simulink model "Neurofeedback_PID_WithoutFNIRS_v1"  (R2021b)
settings: Solver=VariableStepAuto  StartTime=0.0  StopTime=60  FixedStep=0.09  RelTol=1e-10
libraries: slpidlib x1
settings Model: NumberOfSteps=10  SnapshotInterval=100  Creator=mdls3  LastModifiedBy=mdls3
settings SolverCC: ZeroCrossControl=EnableAll
settings DebuggingCC: UnderSpecifiedDimensionMsg=warning

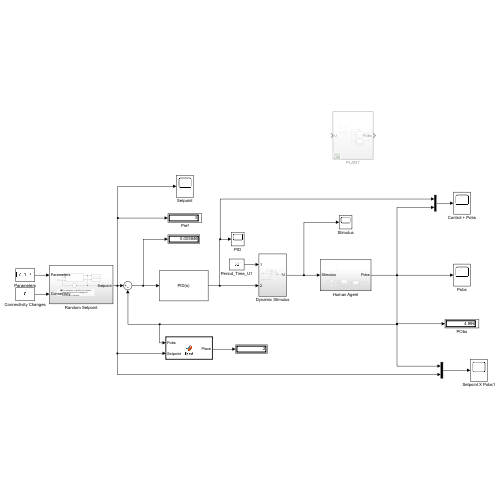
[thumbnail: Simulink's stored preview of the top-level diagram]
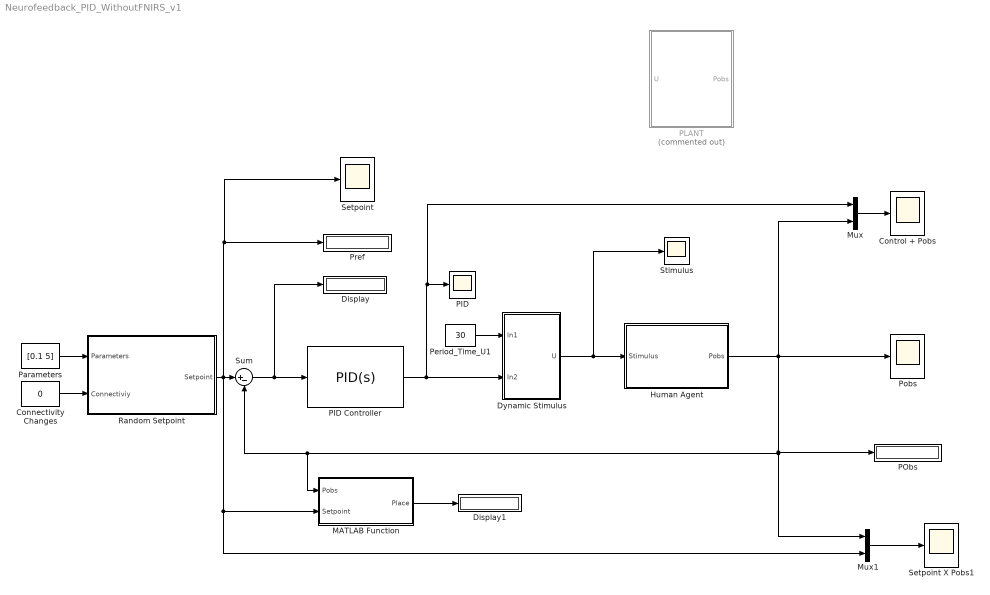
== system Neurofeedback_PID_WithoutFNIRS_v1 ==
  Connectivity Changes : Constant  Value=0
  Control + Pobs : Scope
  Display : Display
  Display1 : Display
  Dynamic Stimulus : Subsystem
  Human Agent : Subsystem
  MATLAB Function : MATLAB Function  TreatAsAtomicUnit=on
  Mux : Mux  Inputs=2
  Mux1 : Mux  Inputs=2
  PID : Scope
  PID Controller : slpidlib/PID Controller  Controller=PID  Form=Ideal  TimeDomain=Continuous-time  UseExternalTs=off  SampleTime=-1  IntegratorMethod=Forward Euler  FilterMethod=Forward Euler  ControllerParametersSource=internal  P=0.6  I=0.075  D=0.015  UseFilter=on  N=100  TunerSelectOption=Transfer Function Based (PID Tuner App)  InitialConditionSource=internal  InitialConditionForIntegrator=1  InitialConditionForFilter=0  DifferentiatorICPrevScaledInput=0  ExternalReset=none  TrackingMode=off  Kt=1  LimitOutput=off  SatLimitsSource=internal  UpperSaturationLimit=inf  LowerSaturationLimit=-inf  LinearizeAsGain=on  AntiWindupMode=none  Kb=1  POutMin=[]  POutMax=[]  IOutMin=[]  IOutMax=[]  DOutMin=[]  DOutMax=[]  NOutMin=[]  NOutMax=[]  SumOutMin=[]  SumOutMax=[]  SaturationOutMin=[]  SaturationOutMax=[]  PParamMin=[]  PParamMax=[]  IParamMin=[]  IParamMax=[]  DParamMin=[]  DParamMax=[]  NParamMin=[]  NParamMax=[]  KbParamMin=[]  KbParamMax=[]  KtParamMin=[]  KtParamMax=[]  KbOutMin=[]  KbOutMax=[]  KtOutMin=[]  KtOutMax=[]  IntegratorOutMin=[]  IntegratorOutMax=[]  FilterOutMin=[]  FilterOutMax=[]  SumI1OutMin=[]  SumI1OutMax=[]  SumI2OutMin=[]  SumI2OutMax=[]  SumI3OutMin=[]  SumI3OutMax=[]  SumI4OutMin=[]  SumI4OutMax=[]  SumDOutMin=[]  SumDOutMax=[]  DifferentiatorOutMin=[]  DifferentiatorOutMax=[]  FilterDiffOutCoefMin=[]  FilterDiffOutCoefMax=[]  ReciprocalOutMin=[]  ReciprocalOutMax=[]  SumDenOutMin=[]  SumDenOutMax=[]  SumNumOutMin=[]  SumNumOutMax=[]  DivideOutMin=[]  DivideOutMax=[]  UdiffTsProdOutMin=[]  UdiffTsProdOutMax=[]  NTsProdOutMin=[]  NTsProdOutMax=[]  UintegralTsProdOutMin=[]  UintegralTsProdOutMax=[]  UngainTsProdOutMin=[]  UngainTsProdOutMax=[]  IntegratorContinuousStateAttributes=''  IntegratorStateMustResolveToSignalObject=off  IntegratorRTWStateStorageClass=Auto  FilterContinuousStateAttributes=''  FilterStateMustResolveToSignalObject=off  FilterRTWStateStorageClass=Auto  ParallelPVariant=Passthrough  IdealPVariant=InternalParameters  IVariant=InternalParameters  DVariant=InternalParameters  IntegratorVariant=Continuous  SatVariant=Disabled  AWVariant=Passthrough  PCopyVariant=Disabled  TRVariant=Disabled  FdbkBlocksVariant=Forward  IdealPFdbkVariant=Disabled  SatFdbkVariant=Disabled  DerivativeFilterVariant=ContFilter  NVariant=InternalParameters  NCopyVariant=Disabled  FilterICVariant=InternalICsFilter  IntegratorICVariant=InternalICs  ExternalResetVariant=Disabled  TRSumVariant=Passthrough  SumFdbkVariant=Disabled  SumVariant=Sum_PID  TsampFilterVariant=InternalTs  TsampNgainVariant=Passthrough  TsampIntegralVariant=Passthrough  ExternalSaturationOutDataTypeStr=Inherit: Same as second input
  PLANT : Subsystem  Commented=on
  PObs : Display
  Parameters : Constant  Value=[0.1 5]
  Period_Time_U1 : Constant  Value=30
  Pobs : Scope
  Pref : Display
  Random Setpoint : Subsystem
  Setpoint : Scope
  Setpoint X Pobs1 : Scope
  Stimulus : Scope
  Sum : Sum  Inputs=|+-
  wires:
  Period_Time_U1/1 -> Dynamic Stimulus/1(In1)
  Dynamic Stimulus/1(U) -> Stimulus/1, Human Agent/1(Stimulus)
  PID Controller/1 -> Dynamic Stimulus/2(In2), Mux/1, PID/1
  Sum/1 -> PID Controller/1, Display/1
  Human Agent/1(Pobs) -> Mux1/1, MATLAB Function/1(Pobs), Sum/2, PObs/1, Pobs/1, Mux/2
  Parameters/1 -> Random Setpoint/1(Parameters)
  Random Setpoint/1(Setpoint) -> MATLAB Function/2(Setpoint), Mux1/2, Setpoint/1, Pref/1, Sum/1
  Connectivity Changes/1 -> Random Setpoint/2(Connectiviy)
  Mux/1 -> Control + Pobs/1
  Mux1/1 -> Setpoint X Pobs1/1
  MATLAB Function/1(Place) -> Display1/1

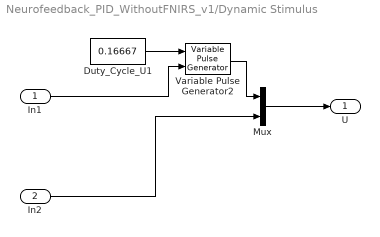
== system Neurofeedback_PID_WithoutFNIRS_v1/Dynamic Stimulus ==
  In1 : Inport
  In2 : Inport  Port=2
  Duty_Cycle_U1 : Constant  Value=0.16667  OutMin=[0]  OutMax=[0.8]
  Mux : Mux  Inputs=2
  Variable Pulse Generator2 : VariablePulseGenerator  RunAtFixedTimeIntervals=on  SampleTime=1/10.4
  U : Outport
  wires:
  In1/1 -> Variable Pulse Generator2/2
  Mux/1 -> U/1
  Variable Pulse Generator2/1 -> Mux/1
  Duty_Cycle_U1/1 -> Variable Pulse Generator2/1
  In2/1 -> Mux/2

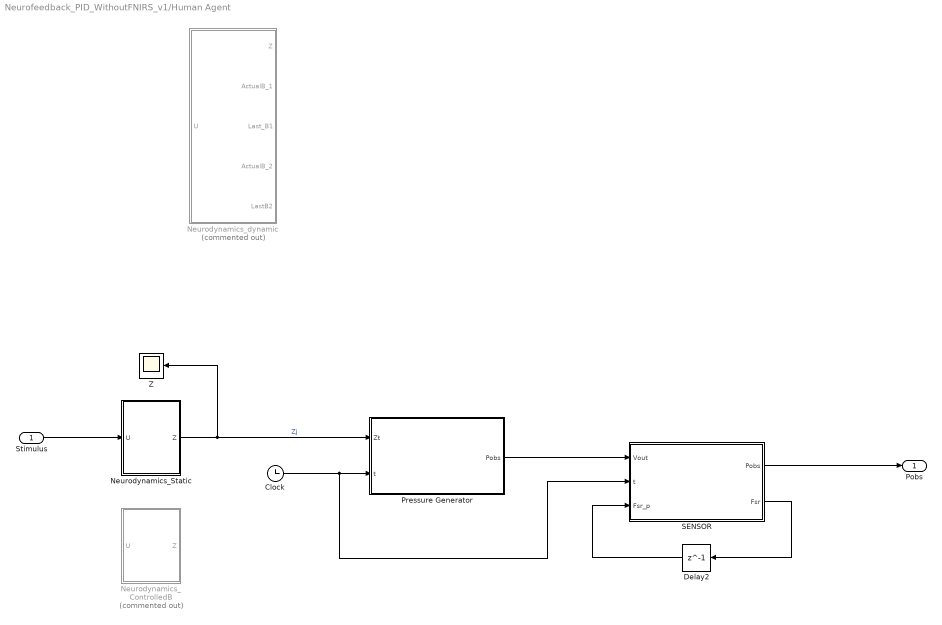
== system Neurofeedback_PID_WithoutFNIRS_v1/Human Agent ==
  Stimulus : Inport
  Clock : Clock
  Delay2 : Delay  DelayLength=1  InitialCondition=0.0001
  Neurodynamics_ControlledB : Subsystem  Commented=on
  "Neurodynamics_Static " : Subsystem
  Neurodynamics_dynamic : Subsystem  Commented=on
  Pressure Generator : MATLAB Function  TreatAsAtomicUnit=on
  SENSOR : MATLAB Function  TreatAsAtomicUnit=on
  Z : Scope
  Pobs : Outport
  wires:
  Pressure Generator/1(Pobs) -> SENSOR/1(Vout)
  Delay2/1 -> SENSOR/3(Fsr_p)
  SENSOR/2(Fsr) -> Delay2/1
  SENSOR/1(Pobs) -> Pobs/1
  Clock/1 -> Pressure Generator/2(t), SENSOR/2(t)
  "Neurodynamics_Static "/1(Z) -> Pressure Generator/1(Zt), Z/1  "Zj"
  Stimulus/1 -> "Neurodynamics_Static "/1(U)

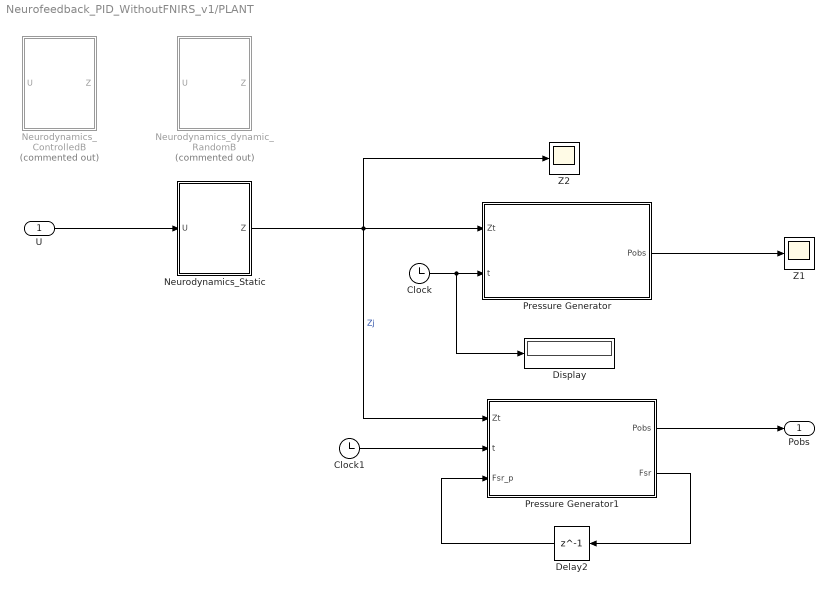
== system Neurofeedback_PID_WithoutFNIRS_v1/PLANT ==
  U : Inport
  Clock : Clock
  Clock1 : Clock
  Delay2 : Delay  DelayLength=1  InitialCondition=0.0001
  Display : Display
  Neurodynamics_ControlledB : Subsystem  Commented=on
  "Neurodynamics_Static " : Subsystem
  Neurodynamics_dynamic_RandomB : Subsystem  Commented=on
  Pressure Generator : MATLAB Function  TreatAsAtomicUnit=on
  Pressure Generator1 : MATLAB Function  TreatAsAtomicUnit=on
  Z1 : Scope
  Z2 : Scope
  Pobs : Outport
  wires:
  Clock/1 -> Display/1, Pressure Generator/2(t)
  Clock1/1 -> Pressure Generator1/2(t)
  Pressure Generator1/2(Fsr) -> Delay2/1
  Pressure Generator1/1(Pobs) -> Pobs/1
  Delay2/1 -> Pressure Generator1/3(Fsr_p)
  Pressure Generator/1(Pobs) -> Z1/1
  "Neurodynamics_Static "/1(Z) -> Pressure Generator1/1(Zt), Z2/1, Pressure Generator/1(Zt)  "Zj"
  U/1 -> "Neurodynamics_Static "/1(U)

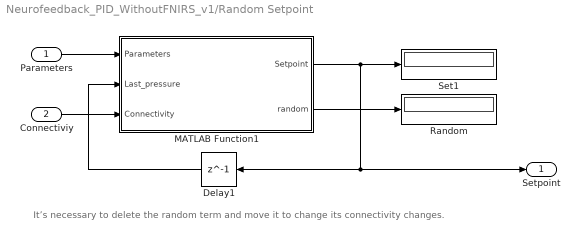
== system Neurofeedback_PID_WithoutFNIRS_v1/Random Setpoint ==
  note: It’s necessary to delete the random term and move it to change its connectivity changes.
  Parameters : Inport
  Connectiviy : Inport  Port=2
  Delay1 : Delay  DelayLength=1  InitialCondition=0
  MATLAB Function1 : MATLAB Function  TreatAsAtomicUnit=on
  Random : Display
  Set1 : Display
  Setpoint : Outport
  wires:
  Parameters/1 -> MATLAB Function1/1(Parameters)
  MATLAB Function1/2(random) -> Random/1
  MATLAB Function1/1(Setpoint) -> Set1/1, Setpoint/1, Delay1/1
  Delay1/1 -> MATLAB Function1/2(Last_pressure)
  Connectiviy/1 -> MATLAB Function1/3(Connectivity)

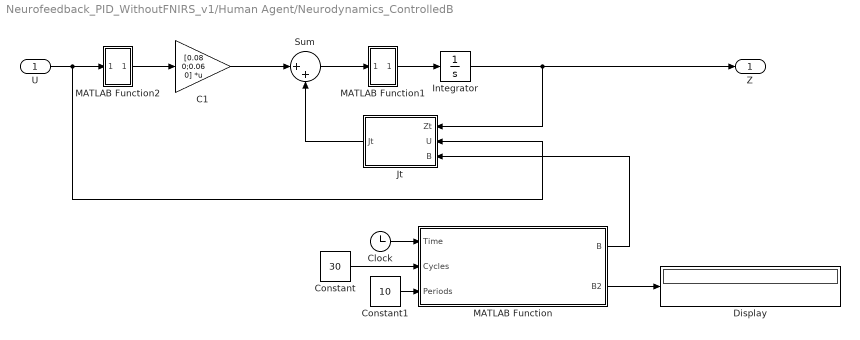
== system Neurofeedback_PID_WithoutFNIRS_v1/Human Agent/Neurodynamics_ControlledB ==
  U : Inport
  C1 : Gain  Gain=[0.08 0;0.06 0]  Multiplication=Matrix(K*u) (u vector)
  Clock : Clock
  Constant : Constant  Value=30
  Constant1 : Constant  Value=10
  Display : Display
  Integrator : Integrator
  Jt : MATLAB Function  TreatAsAtomicUnit=on
  MATLAB Function : MATLAB Function  TreatAsAtomicUnit=on
  MATLAB Function1 : MATLAB Function  TreatAsAtomicUnit=on
  MATLAB Function2 : MATLAB Function  TreatAsAtomicUnit=on
  Sum : Sum  Inputs=|++
  Z : Outport
  wires:
  Jt/1(Jt) -> Sum/2
  U/1 -> MATLAB Function2/1(Z), Jt/2(U)
  Constant1/1 -> MATLAB Function/3(Periods)
  Clock/1 -> MATLAB Function/1(Time)
  Constant/1 -> MATLAB Function/2(Cycles)
  MATLAB Function/2(B2) -> Display/1
  MATLAB Function/1(B) -> Jt/3(B)
  Integrator/1 -> Z/1, Jt/1(Zt)
  MATLAB Function1/1(Zn) -> Integrator/1
  Sum/1 -> MATLAB Function1/1(Z)
  MATLAB Function2/1(Zn) -> C1/1
  C1/1 -> Sum/1

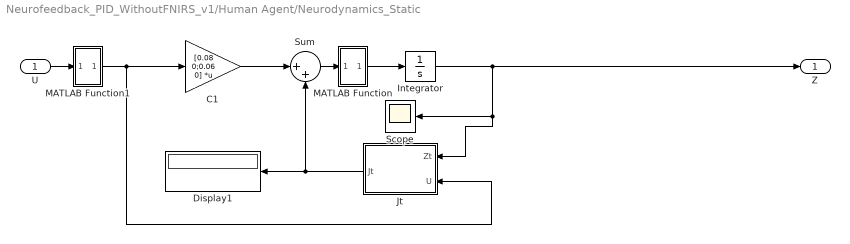
== system Neurofeedback_PID_WithoutFNIRS_v1/Human Agent/Neurodynamics_Static  ==
  U : Inport
  C1 : Gain  Gain=[0.08 0;0.06 0]  Multiplication=Matrix(K*u) (u vector)
  Display1 : Display
  Integrator : Integrator
  Jt : MATLAB Function  TreatAsAtomicUnit=on
  MATLAB Function : MATLAB Function  TreatAsAtomicUnit=on
  MATLAB Function1 : MATLAB Function  TreatAsAtomicUnit=on
  Scope : Scope
  Sum : Sum  Inputs=|++
  Z : Outport
  wires:
  Integrator/1 -> Z/1, Scope/1, Jt/1(Zt)
  C1/1 -> Sum/1
  Jt/1(Jt) -> Sum/2, Display1/1
  U/1 -> MATLAB Function1/1(Z)
  Sum/1 -> MATLAB Function/1(Z)
  MATLAB Function1/1(Zn) -> C1/1, Jt/2(U)
  MATLAB Function/1(Zn) -> Integrator/1

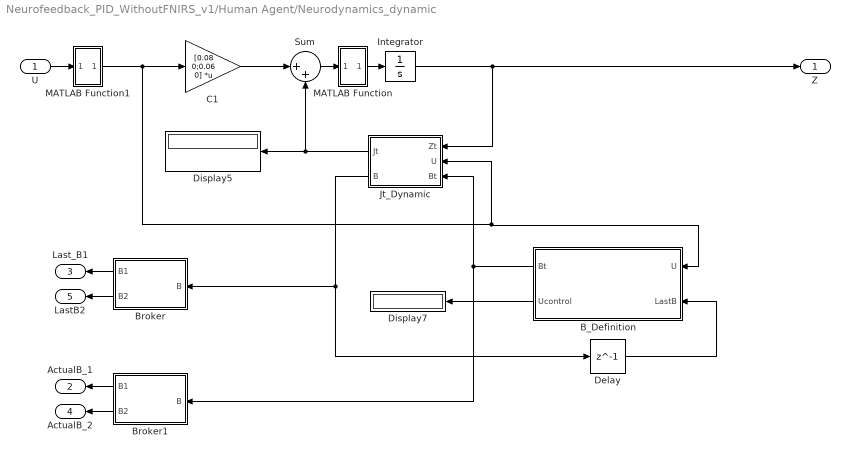
== system Neurofeedback_PID_WithoutFNIRS_v1/Human Agent/Neurodynamics_dynamic ==
  U : Inport
  B_Definition : MATLAB Function  TreatAsAtomicUnit=on
  Broker : MATLAB Function  TreatAsAtomicUnit=on
  Broker1 : MATLAB Function  TreatAsAtomicUnit=on
  C1 : Gain  Gain=[0.08 0;0.06 0]  Multiplication=Matrix(K*u) (u vector)
  Delay : Delay  DelayLength=1  InitialCondition=0
  Display5 : Display
  Display7 : Display
  Integrator : Integrator
  Jt_Dynamic : MATLAB Function  TreatAsAtomicUnit=on
  MATLAB Function : MATLAB Function  TreatAsAtomicUnit=on
  MATLAB Function1 : MATLAB Function  TreatAsAtomicUnit=on
  Sum : Sum  Inputs=|++
  Z : Outport
  ActualB_1 : Outport  Port=2
  Last_B1 : Outport  Port=3
  ActualB_2 : Outport  Port=4
  LastB2 : Outport  Port=5
  wires:
  Integrator/1 -> Z/1, Jt_Dynamic/1(Zt)
  C1/1 -> Sum/1
  U/1 -> MATLAB Function1/1(Z)
  Sum/1 -> MATLAB Function/1(Z)
  MATLAB Function1/1(Zn) -> C1/1, B_Definition/1(U), Jt_Dynamic/2(U)
  MATLAB Function/1(Zn) -> Integrator/1
  Jt_Dynamic/1(Jt) -> Display5/1, Sum/2
  Delay/1 -> B_Definition/2(LastB)
  Jt_Dynamic/2(B) -> Broker/1(B), Delay/1
  B_Definition/1(Bt) -> Jt_Dynamic/3(Bt), Broker1/1(B)
  B_Definition/2(Ucontrol) -> Display7/1
  Broker1/1(B1) -> ActualB_1/1
  Broker1/2(B2) -> ActualB_2/1
  Broker/2(B2) -> LastB2/1
  Broker/1(B1) -> Last_B1/1

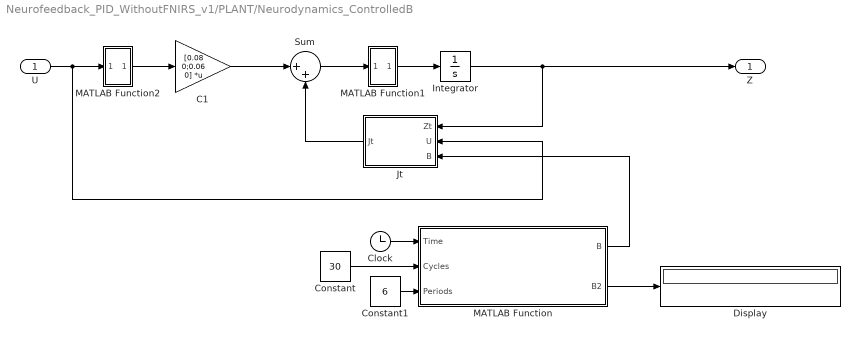
== system Neurofeedback_PID_WithoutFNIRS_v1/PLANT/Neurodynamics_ControlledB ==
  U : Inport
  C1 : Gain  Gain=[0.08 0;0.06 0]  Multiplication=Matrix(K*u) (u vector)
  Clock : Clock
  Constant : Constant  Value=30
  Constant1 : Constant  Value=6
  Display : Display
  Integrator : Integrator
  Jt : MATLAB Function  TreatAsAtomicUnit=on
  MATLAB Function : MATLAB Function  TreatAsAtomicUnit=on
  MATLAB Function1 : MATLAB Function  TreatAsAtomicUnit=on
  MATLAB Function2 : MATLAB Function  TreatAsAtomicUnit=on
  Sum : Sum  Inputs=|++
  Z : Outport
  wires:
  Jt/1(Jt) -> Sum/2
  U/1 -> MATLAB Function2/1(Z), Jt/2(U)
  Constant1/1 -> MATLAB Function/3(Periods)
  Clock/1 -> MATLAB Function/1(Time)
  Constant/1 -> MATLAB Function/2(Cycles)
  MATLAB Function/2(B2) -> Display/1
  MATLAB Function/1(B) -> Jt/3(B)
  Integrator/1 -> Z/1, Jt/1(Zt)
  MATLAB Function1/1(Zn) -> Integrator/1
  Sum/1 -> MATLAB Function1/1(Z)
  MATLAB Function2/1(Zn) -> C1/1
  C1/1 -> Sum/1

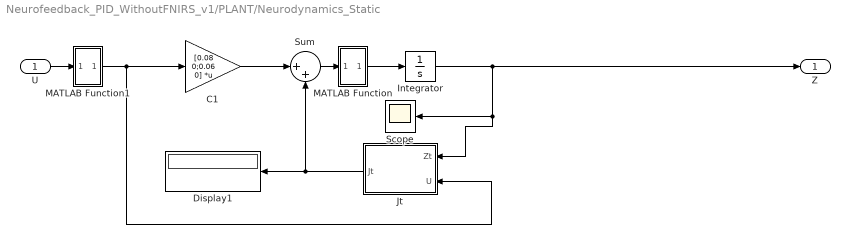
== system Neurofeedback_PID_WithoutFNIRS_v1/PLANT/Neurodynamics_Static  ==
  U : Inport
  C1 : Gain  Gain=[0.08 0;0.06 0]  Multiplication=Matrix(K*u) (u vector)
  Display1 : Display
  Integrator : Integrator
  Jt : MATLAB Function  TreatAsAtomicUnit=on
  MATLAB Function : MATLAB Function  TreatAsAtomicUnit=on
  MATLAB Function1 : MATLAB Function  TreatAsAtomicUnit=on
  Scope : Scope
  Sum : Sum  Inputs=|++
  Z : Outport
  wires:
  Integrator/1 -> Z/1, Scope/1, Jt/1(Zt)
  C1/1 -> Sum/1
  Jt/1(Jt) -> Sum/2, Display1/1
  U/1 -> MATLAB Function1/1(Z)
  Sum/1 -> MATLAB Function/1(Z)
  MATLAB Function1/1(Zn) -> C1/1, Jt/2(U)
  MATLAB Function/1(Zn) -> Integrator/1

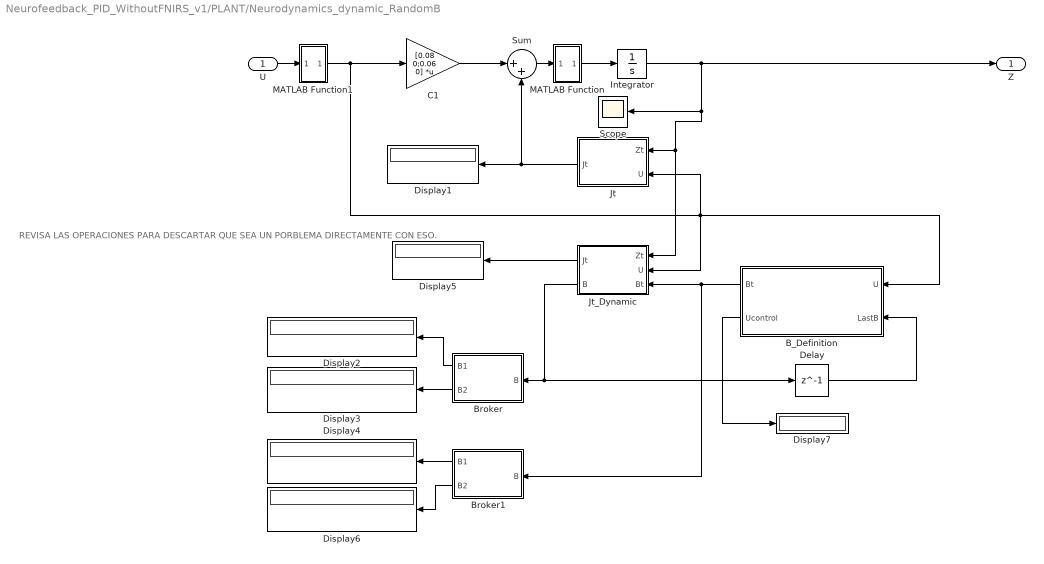
== system Neurofeedback_PID_WithoutFNIRS_v1/PLANT/Neurodynamics_dynamic_RandomB ==
  note: REVISA LAS OPERACIONES PARA DESCARTAR QUE SEA UN PORBLEMA DIRECTAMENTE CON ESO.
  U : Inport
  B_Definition : MATLAB Function  TreatAsAtomicUnit=on
  Broker : MATLAB Function  TreatAsAtomicUnit=on
  Broker1 : MATLAB Function  TreatAsAtomicUnit=on
  C1 : Gain  Gain=[0.08 0;0.06 0]  Multiplication=Matrix(K*u) (u vector)
  Delay : Delay  DelayLength=1  InitialCondition=0
  Display{1..7} (7 alike) : Display
  Integrator : Integrator
  Jt : MATLAB Function  TreatAsAtomicUnit=on
  Jt_Dynamic : MATLAB Function  TreatAsAtomicUnit=on
  MATLAB Function : MATLAB Function  TreatAsAtomicUnit=on
  MATLAB Function1 : MATLAB Function  TreatAsAtomicUnit=on
  Scope : Scope
  Sum : Sum  Inputs=|++
  Z : Outport
  wires:
  Integrator/1 -> Z/1, Scope/1, Jt/1(Zt), Jt_Dynamic/1(Zt)
  C1/1 -> Sum/1
  Jt/1(Jt) -> Sum/2, Display1/1
  U/1 -> MATLAB Function1/1(Z)
  Sum/1 -> MATLAB Function/1(Z)
  MATLAB Function1/1(Zn) -> C1/1, Jt/2(U), B_Definition/1(U), Jt_Dynamic/2(U)
  MATLAB Function/1(Zn) -> Integrator/1
  Jt_Dynamic/1(Jt) -> Display5/1
  Delay/1 -> B_Definition/2(LastB)
  Jt_Dynamic/2(B) -> Broker/1(B), Delay/1
  Broker/1(B1) -> Display2/1
  Broker/2(B2) -> Display3/1
  B_Definition/1(Bt) -> Broker1/1(B), Jt_Dynamic/3(Bt)
  Broker1/2(B2) -> Display6/1
  Broker1/1(B1) -> Display4/1
  B_Definition/2(Ucontrol) -> Display7/1

== matlab function Neurofeedback_PID_WithoutFNIRS_v1/PLANT/Neurodynamics_dynamic_RandomB/Jt ==
  data: Zt input; U input; Jt output
function Jt = fcn(Zt, U)
   A = [-0.16 -0.49;-0.02 -0.33];
   nRegions  = size(A,1);
   M = size(U,1); %nStimuli
   simulationLength = size(U,2);
   B = zeros(2,2,2);
   B1 = [0 0; 0 0]; %There must be a B per stimulus
   B2 = [-0.02 -0.77; 0.33 -1.31];
   B(:,:,1) = B1;
   B(:,:,2) = B2;
      assert(M == size(B,3),...
       'Unexpected number of induced connectivity parameters B.');
   T = zeros(nRegions); %nRegions x nRegions
    for t = 1:simulationLength
           for uu = 1:M % Sum (Uj * Bj)
               tmp = U(uu,t)*B(:,:,uu);
               T = -0.5*exp(T + tmp);  
           end
    end
    SI = diag(A);
    A =  A - diag(exp(SI) + (SI));
Jt = (A*Zt) + (T*Zt);

== matlab function Neurofeedback_PID_WithoutFNIRS_v1/PLANT/Neurodynamics_ControlledB/Jt ==
  data: Zt input; U input; Jt output; B input
function Jt = fcn(Zt, U,B)
   A = [-0.16 -0.49;-0.02 -0.33];
   nRegions  = size(A,1);
   M = size(U,1); %nStimuli
   simulationLength = size(U,2);
%    B = zeros(2,2,2);
%    B1 = [0 0; 0 0]; %There must be a B per stimulus
%    %B2_3
%    B2 = [-0.67 -0.91 ;-0.3 -1.21];
%    %B2_2
%    %B2 = [-0.08 -1.08; 1.2054 -0.0076];
%    %B2_1
%    %B2 = [-0.02 -0.07; 0.33 -1.31];
%    B(:,:,1) = B1;
%    B(:,:,2) = B2;
      assert(M == size(B,3),...
       'Unexpected number of induced connectivity parameters B.');
   T = zeros(nRegions); %nRegions x nRegions
    for t = 1:simulationLength
           for uu = 1:M % Sum (Uj * Bj)
               tmp = U(uu,t)*B(:,:,uu);
               T = -0.5*exp(T + tmp);  
           end
    end
    SI = diag(A);
    A =  A - diag(exp(SI) + (SI));
Jt = (A*Zt) + (T*Zt);

== matlab function Neurofeedback_PID_WithoutFNIRS_v1/PLANT/Neurodynamics_dynamic_RandomB/MATLAB Function ==
  data: Z input; Zn output
function Zn = fcn(Z)

Zn = Z(:,1);

== matlab function Neurofeedback_PID_WithoutFNIRS_v1/PLANT/Neurodynamics_dynamic_RandomB/MATLAB Function1 ==
  data: Z input; Zn output
function Zn = fcn(Z)

Zn = Z(:,1);

== matlab function Neurofeedback_PID_WithoutFNIRS_v1/Human Agent/Neurodynamics_Static /Jt ==
  data: Zt input; U input; Jt output
function Jt = fcn(Zt, U)
   A = [-0.16 -0.49;-0.02 -0.33];
   nRegions  = size(A,1);
   M = size(U,1); %nStimuli
   simulationLength = size(U,2);
   B = zeros(2,2,2);
   B1 = [0 0; 0 0]; %There must be a B per stimulus
   B2 = [-0.02 -0.77; 0.33 -1.31];
   B(:,:,1) = B1;
   B(:,:,2) = B2;
      assert(M == size(B,3),...
       'Unexpected number of induced connectivity parameters B.');
   T = zeros(nRegions); %nRegions x nRegions
    for t = 1:simulationLength
           for uu = 1:M % Sum (Uj * Bj)
               tmp = U(uu,t)*B(:,:,uu);
               T = -0.5*exp(T + tmp);  
           end
    end
    SI = diag(A);
    A =  A - diag(exp(SI) + (SI));
Jt = (A*Zt) + (T*Zt);

== matlab function Neurofeedback_PID_WithoutFNIRS_v1/PLANT/Pressure Generator ==
  data: Zt input; Pobs output; t input
function Pobs = fcn(Zt, t)
    R=10000; %Resistor [Ohms];
    C=0.1; %Capacitor [Faradays];
    V= Zt(1,:); %Voltage or system reference;
    Vc = V * (1 - exp(-t/(R*C))); % Voltage at the capacitor  
    
Pobs = Vc;

== matlab function Neurofeedback_PID_WithoutFNIRS_v1/Human Agent/Neurodynamics_Static /MATLAB Function ==
  data: Z input; Zn output
function Zn = fcn(Z)

Zn = Z(:,1);

== matlab function Neurofeedback_PID_WithoutFNIRS_v1/Human Agent/Neurodynamics_Static /MATLAB Function1 ==
  data: Z input; Zn output
function Zn = fcn(Z)

Zn = Z(:,1);

== matlab function Neurofeedback_PID_WithoutFNIRS_v1/PLANT/Neurodynamics_Static /Jt ==
  data: Zt input; U input; Jt output
function Jt = fcn(Zt, U)
   A = [-0.16 -0.49;-0.02 -0.33];
   nRegions  = size(A,1);
   M = size(U,1); %nStimuli
   simulationLength = size(U,2);
   B = zeros(2,2,2);
   B1 = [0 0; 0 0]; %There must be a B per stimulus
   B2 = [-0.02 -0.77; 0.33 -1.31];
   B(:,:,1) = B1;
   B(:,:,2) = B2;
      assert(M == size(B,3),...
       'Unexpected number of induced connectivity parameters B.');
   T = zeros(nRegions); %nRegions x nRegions
    for t = 1:simulationLength
           for uu = 1:M % Sum (Uj * Bj)
               tmp = U(uu,t)*B(:,:,uu);
               T = -0.5*exp(T + tmp);  
           end
    end
    SI = diag(A);
    A =  A - diag(exp(SI) + (SI));
Jt = (A*Zt) + (T*Zt);

== matlab function Neurofeedback_PID_WithoutFNIRS_v1/Human Agent/Neurodynamics_ControlledB/MATLAB Function ==
  settings: updateMethod=DISCRETE
  data: Time input; B output; Cycles input; Periods input; B2 output
function [B, B2] = ControlledDynamic_B(Time, Cycles, Periods)

   B = zeros(2,2,2);
   %B1 = [0 0; 0 0]; %There must be a B per stimulus
   %B2_3
   %B2 = [-0.67 -0.91 ;-0.3 -1.21];
   %B2_2
   %B2 = [-0.08 -1.08; 1.2054 -0.0076];
   %B2_1
   %B2 = [-0.02 -0.07; 0.33 -1.31];
   PCycles = zeros(10,1);
   for i = 1:Periods
       PCycles(i) = i * Cycles;   
   end
   %random_selector = randi([1,3]);

   if(Time >= 0 && Time <= PCycles(2))
%       random_selector = randi([1,3]);
%       if(random_selector == 1)
          B1 = [0 0; 0 0];
          B2 = [-0.02 -0.07; 0.33 -1.31]; 
%       elseif(random_selector == 2)
%           B1 = [0 0; 0 0];
%           B2 = [-0.08 -1.08; 1.2054 -0.0076];
%       else
%           B1 = [0 0; 0 0];
%           B2 = [-0.67 -0.91; 0.3 -1.21];
      B(:,:,1) = B1;
      B(:,:,2) = B2;
   elseif(Time >= PCycles(2)+1 && Time <= PCycles(4))
       B1 = [0 0;0 0];
       B2 = [-0.08 -1.08; 1.2054 -0.0076];
       B(:,:,1) = B1;
       B(:,:,2) = B2;
   else
       B1 = [0 0; 0 0];
       B2 = [-0.67 -0.91; -0.3 -1.21];
       B(:,:,1) = B1;
       B(:,:,2) = B2;
   end

== matlab function Neurofeedback_PID_WithoutFNIRS_v1/PLANT/Neurodynamics_Static /MATLAB Function ==
  data: Z input; Zn output
function Zn = fcn(Z)

Zn = Z(:,1);

== matlab function Neurofeedback_PID_WithoutFNIRS_v1/PLANT/Neurodynamics_Static /MATLAB Function1 ==
  data: Z input; Zn output
function Zn = fcn(Z)

Zn = Z(:,1);

== matlab function Neurofeedback_PID_WithoutFNIRS_v1/MATLAB Function ==
  data: Pobs input; Place output; Setpoint input
function Place = feed(Pobs, Setpoint)
    
    %Sensor maximum limit 
    Range = 10;
    Limit =  (Range - Setpoint)/2;
    temp = 0;
    Nm = (Setpoint - Limit);
    Nl = (Setpoint - Limit)*2;
    
    Pl = (Setpoint + Limit);
    Pm = (Setpoint + Limit)*2;
    
    if ((Pobs > Pl) && (Pobs < Pm))
        temp = 4;
    elseif((Pobs > Setpoint) && (Pobs < Pl))
        temp = 3;
    elseif((Pobs > Nm) && (Pobs < Setpoint))
        temp = 2;
    else
        temp = 1;

    end
    
    Place = temp;

== matlab function Neurofeedback_PID_WithoutFNIRS_v1/Human Agent/Neurodynamics_dynamic/B_Definition ==
  settings: updateMethod=DISCRETE
  data: U input; Bt output; LastB input; Ucontrol output
function [Bt, Ucontrol] = B_Definition(U, LastB)
   Bt = zeros(2, 2, 2);
   %Control extraction and weight
   Ucontrol = U(2) * (0.2 + rand(1) * (1-0.2));
   Threshold = 0.2;
    if(Ucontrol < Threshold) %Random Ucontrol to test
        min = -1; 
        max = 1.5;
        n = 2;
        r1 = min + rand(n)*(max-min);
        r2 = min + rand(n)*(max-min);
        %Bt(:,:,1) = r1(:,:);
        Bt(:,:,2) = r2(:,:);
    else
       Bt = LastB;
    end

== matlab function Neurofeedback_PID_WithoutFNIRS_v1/Human Agent/Neurodynamics_dynamic/Broker ==
  data: B input; B1 output; B2 output
function [B1, B2] = fcn(B)
B1 = B(:,:,1);
B2 = B(:,:,2);

== matlab function Neurofeedback_PID_WithoutFNIRS_v1/Human Agent/Neurodynamics_dynamic/Broker1 ==
  data: B input; B1 output; B2 output
function [B1, B2] = fcn(B)
B1 = B(:,:,1);
B2 = B(:,:,2);

== matlab function Neurofeedback_PID_WithoutFNIRS_v1/Human Agent/Neurodynamics_dynamic/Jt_Dynamic ==
  data: Zt input; U input; Jt output; Bt input; B output
function [Jt, B] = fcn(Zt, U, Bt)

   A = [-0.16 -0.49;-0.02 -0.33];
   nRegions  = size(A,1);

   B = zeros(2,2,2);
   a = 0;
   B1 = [0 0; 0 0]; %There must be a B per stimulus
   B2 = [-0.02 -0.77; 0.33 -1.31];

   if Bt(:,:,2) ~= B(:,:,2)
       B(:,:,:) = Bt(:,:,:);
   else
          B(:,:,1) = B1;
          B(:,:,2) = B2;
   end
   M = size(U,1); %nStimuli
   assert(M == size(B,3),...
        'Unexpected number of induced connectivity parameters B.');

    simulationLength = size(U,2);
    for t = 1:simulationLength
       T = zeros(nRegions); %nRegions x nRegions
                   for uu = 1:M % Sum (Uj * Bj)
                       tmp = U(uu,t) * B(:,:,uu);
                       T = -0.5 * exp(T + tmp);  
                   end
            SI = diag(A);
    end
        A =  A - diag(exp(SI) + (SI));
Jt = (A*Zt) + (T*Zt);

== matlab function Neurofeedback_PID_WithoutFNIRS_v1/Random Setpoint/MATLAB Function1 ==
  settings: updateMethod=DISCRETE
  data: Setpoint output; Parameters input; Last_pressure input; random output; Connectivity input
function [Setpoint, random] = Random_Setpoint(Parameters, Last_pressure, Connectivity)
    %Parameters = [threshold Start_setpoint]
    temp = 0;
   %Pressure Setpoint selection
    pmin = 3;
    pmax = 10;
    new_pressure = pmin + rand(1)*(pmax-pmin);

    %Random used to simulate the connectivity changes, so we must change
    %the pressure setpoint when changes in the connectitvy are observed.
    min = 0;
    tmax = 10;
        %We should fine a random criteria to change the setpoint, not just
        %time, or the moment B changes. For now works to demostrate the
        %control without fNIRS
    random = min + rand(1) * (tmax - min) * new_pressure;
    if (Connectivity == 1)
         if (random < Parameters(1))
            %disp("Time")
            %disp(Time)
            temp = new_pressure;
            %disp("Setpoint")
            %disp(temp)
        else 
            temp = Last_pressure;
                if (Parameters(2) == temp || temp == 0)
                    temp = Parameters(2);
                else
                    temp = Last_pressure;
                end
         end  
    else
        temp = Parameters(2);
    end

    Setpoint = temp;

== matlab function Neurofeedback_PID_WithoutFNIRS_v1/Human Agent/Neurodynamics_dynamic/MATLAB Function ==
  data: Z input; Zn output
function Zn = fcn(Z)

Zn = Z(:,1);

== matlab function Neurofeedback_PID_WithoutFNIRS_v1/Human Agent/Neurodynamics_dynamic/MATLAB Function1 ==
  data: Z input; Zn output
function Zn = fcn(Z)

Zn = Z(:,1);

== matlab function Neurofeedback_PID_WithoutFNIRS_v1/Human Agent/Pressure Generator ==
  data: Zt input; Pobs output; t input
function Pobs = fcn(Zt, t)
    R=100; %Resistor [Ohms];
    C= 2.5; %Capacitor [Faradays];
    V= Zt(1); %Voltage or system reference;
    Vc = V * (exp(-t/(R*C))); % Voltage at the capacitor  
    
Pobs = Vc;

== matlab function Neurofeedback_PID_WithoutFNIRS_v1/Human Agent/SENSOR ==
  data: Vout input; Pobs output; t input; Fsr_p input; Fsr output
function [Pobs,Fsr] = PressureGenerator_sensor(Vout, t,Fsr_p)

    Vcc = 500; %Considering 5V as a real sensor, the value is on mV
    Rf = 100; %Fixed resistor 10k ohms
    kgf = 0.1019716213; % 1N = 0.1019716213 kgf
    Fsr = 0;
    Fsrforce = 0;
    Fsr = (Vcc - Vout * Rf) / Vout;
    FsConductance = 1000000; %Sensor conductance in uOhms
    FsConductance = FsConductance / Fsr;
    if FsConductance <= 1000
        Fsrforce = FsConductance / 80; %Force on Newtons
    else
        Fsrforce = FsConductance - 1000;
        Fsrforce = Fsrforce / 30;
    end
    
Pobs = Fsrforce * kgf;

end

== matlab function Neurofeedback_PID_WithoutFNIRS_v1/Human Agent/Neurodynamics_ControlledB/Jt ==
  data: Zt input; U input; Jt output; B input
function Jt = fcn(Zt, U,B)
   A = [-0.16 -0.49;-0.02 -0.33];
   nRegions  = size(A,1);
   M = size(U,1); %nStimuli
   simulationLength = size(U,2);
%    B = zeros(2,2,2);
%    B1 = [0 0; 0 0]; %There must be a B per stimulus
%    %B2_3
%    B2 = [-0.67 -0.91 ;-0.3 -1.21];
%    %B2_2
%    %B2 = [-0.08 -1.08; 1.2054 -0.0076];
%    %B2_1
%    %B2 = [-0.02 -0.07; 0.33 -1.31];
%    B(:,:,1) = B1;
%    B(:,:,2) = B2;
      assert(M == size(B,3),...
       'Unexpected number of induced connectivity parameters B.');
   T = zeros(nRegions); %nRegions x nRegions
    for t = 1:simulationLength
           for uu = 1:M % Sum (Uj * Bj)
               tmp = U(uu,t)*B(:,:,uu);
               T = -0.5*exp(T + tmp);  
           end
    end
    SI = diag(A);
    A =  A - diag(exp(SI) + (SI));
Jt = (A*Zt) + (T*Zt);

== matlab function Neurofeedback_PID_WithoutFNIRS_v1/Human Agent/Neurodynamics_ControlledB/MATLAB Function1 ==
  data: Z input; Zn output
function Zn = fcn(Z)

Zn = Z(:,1);

== matlab function Neurofeedback_PID_WithoutFNIRS_v1/Human Agent/Neurodynamics_ControlledB/MATLAB Function2 ==
  data: Z input; Zn output
function Zn = fcn(Z)

Zn = Z(:,1);

== matlab function Neurofeedback_PID_WithoutFNIRS_v1/PLANT/Neurodynamics_dynamic_RandomB/Broker ==
  data: B input; B1 output; B2 output
function [B1, B2] = fcn(B)
B1 = B(:,:,1);
B2 = B(:,:,2);

== matlab function Neurofeedback_PID_WithoutFNIRS_v1/PLANT/Pressure Generator1 ==
  data: Zt input; Pobs output; t input; Fsr_p input; Fsr output
function [Pobs,Fsr] = PressureGenerator_sensor(Zt, t,Fsr_p)
    C = 2; % 0.1F
    Vcc = 500; %Considering 5V as a real sensor, the value is on mV
    Rf = 1000; %Fixed resistor 10k ohms
    kgf = 0.1019716213; % 1N = 0.1019716213 kgf
    Fsr = 0;
    Fsrforce = 0;

    Vout = Zt(1) * (1 - exp( -t / C)); %Emulation of the capacitor
    Fsr = (Vcc - Vout * Rf) / Vout;
    FsConductance = 1000000; %Sensor conductance in uOhms
    FsConductance = FsConductance / Fsr;
    if FsConductance <= 1000
        Fsrforce = FsConductance / 80; %Force on Newtons
    else
        Fsrforce = FsConductance - 1000;
        Fsrforce = Fsrforce / 30;
    end
    
Pobs = Fsrforce;

end

== matlab function Neurofeedback_PID_WithoutFNIRS_v1/PLANT/Neurodynamics_ControlledB/MATLAB Function ==
  settings: updateMethod=DISCRETE
  data: Time input; B output; Cycles input; Periods input; B2 output
function [B, B2] = ControlledDynamic_B(Time, Cycles, Periods)

   B = zeros(2,2,2);
   %B1 = [0 0; 0 0]; %There must be a B per stimulus
   %B2_3
   %B2 = [-0.67 -0.91 ;-0.3 -1.21];
   %B2_2
   %B2 = [-0.08 -1.08; 1.2054 -0.0076];
   %B2_1
   %B2 = [-0.02 -0.07; 0.33 -1.31];
   PCycles = zeros(6,1);
   for i = 1:Periods
       PCycles(i) = i * Cycles;   
   end
   %random_selector = randi([1,3]);

   if(Time >= 0 && Time <= PCycles(2))
%       random_selector = randi([1,3]);
%       if(random_selector == 1)
          B1 = [0 0; 0 0];
          B2 = [-0.02 -0.07; 0.33 -1.31]; 
%       elseif(random_selector == 2)
%           B1 = [0 0; 0 0];
%           B2 = [-0.08 -1.08; 1.2054 -0.0076];
%       else
%           B1 = [0 0; 0 0];
%           B2 = [-0.67 -0.91; 0.3 -1.21];
      B(:,:,1) = B1;
      B(:,:,2) = B2;
   elseif(Time >= PCycles(2)+1 && Time <= PCycles(4))
       B1 = [0 0;0 0];
       B2 = [-0.08 -1.08; 1.2054 -0.0076];
       B(:,:,1) = B1;
       B(:,:,2) = B2;
   else
       B1 = [0 0; 0 0];
       B2 = [-0.67 -0.91; -0.3 -1.21];
       B(:,:,1) = B1;
       B(:,:,2) = B2;
   end

== matlab function Neurofeedback_PID_WithoutFNIRS_v1/PLANT/Neurodynamics_dynamic_RandomB/Broker1 ==
  data: B input; B1 output; B2 output
function [B1, B2] = fcn(B)
B1 = B(:,:,1);
B2 = B(:,:,2);

== matlab function Neurofeedback_PID_WithoutFNIRS_v1/PLANT/Neurodynamics_ControlledB/MATLAB Function1 ==
  data: Z input; Zn output
function Zn = fcn(Z)

Zn = Z(:,1);

== matlab function Neurofeedback_PID_WithoutFNIRS_v1/PLANT/Neurodynamics_ControlledB/MATLAB Function2 ==
  data: Z input; Zn output
function Zn = fcn(Z)

Zn = Z(:,1);

== matlab function Neurofeedback_PID_WithoutFNIRS_v1/PLANT/Neurodynamics_dynamic_RandomB/Jt_Dynamic ==
  data: Zt input; U input; Jt output; Bt input; B output
function [Jt, B] = fcn(Zt, U, Bt)

   A = [-0.16 -0.49;-0.02 -0.33];
   nRegions  = size(A,1);

   B = zeros(2,2,2);
   a = 0;
   B1 = [0 0; 0 0]; %There must be a B per stimulus
   B2 = [-0.02 -0.77; 0.33 -1.31];

   if Bt(:,:,2) ~= B(:,:,2)
       B(:,:,:) = Bt(:,:,:);
   else
          B(:,:,1) = B1;
          B(:,:,2) = B2;
   end
   M = size(U,1); %nStimuli
   assert(M == size(B,3),...
        'Unexpected number of induced connectivity parameters B.');

    simulationLength = size(U,2);
    for t = 1:simulationLength
       T = zeros(nRegions); %nRegions x nRegions
                   for uu = 1:M % Sum (Uj * Bj)
                       tmp = U(uu,t) * B(:,:,uu);
                       T = -0.5 * exp(T + tmp);  
                   end
            SI = diag(A);
    end
        A =  A - diag(exp(SI) + (SI));
Jt = (A*Zt) + (T*Zt);

== matlab function Neurofeedback_PID_WithoutFNIRS_v1/PLANT/Neurodynamics_dynamic_RandomB/B_Definition ==
  settings: updateMethod=DISCRETE
  data: U input; Bt output; LastB input; Ucontrol output
function [Bt, Ucontrol] = B_Definition(U, LastB)
    Bt = zeros(2, 2, 2);
   %Control extraction and weight
   Ucontrol = U(2) * (0.1 + rand(1) * (1-0.1));
   Threshold = 0.5;
    if(Ucontrol < Threshold) %Random Ucontrol to test
        min = -1.5; 
        max =0.5;
        n = 2;
        r1 = min + rand(n)*(max-min);
        r2 = min + rand(n)*(max-min);
        %Bt(:,:,1) = r1(:,:);
        Bt(:,:,2) = r2(:,:);
    else
       Bt = LastB;
    end
